simulink model "ControlMotor"  (R2024b)
settings: Solver=VariableStepAuto  StartTime=0.0  StopTime=inf  RelTol=1e-3
model workspace (MAT data in the model file):
  Speed = [255 255]
libraries: arduinolib x4
settings Model: Creator=m4ttn  LastModifiedBy=m4ttn

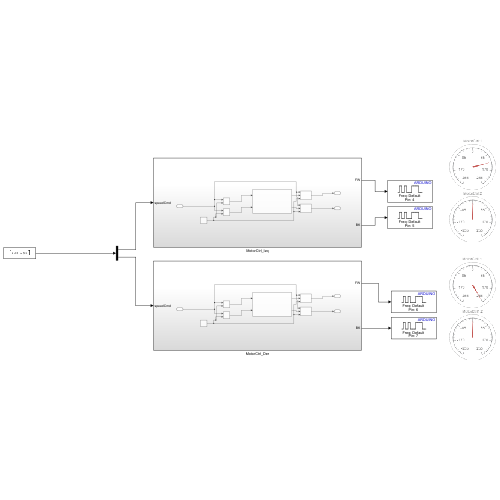
[thumbnail: Simulink's stored preview of the top-level diagram]
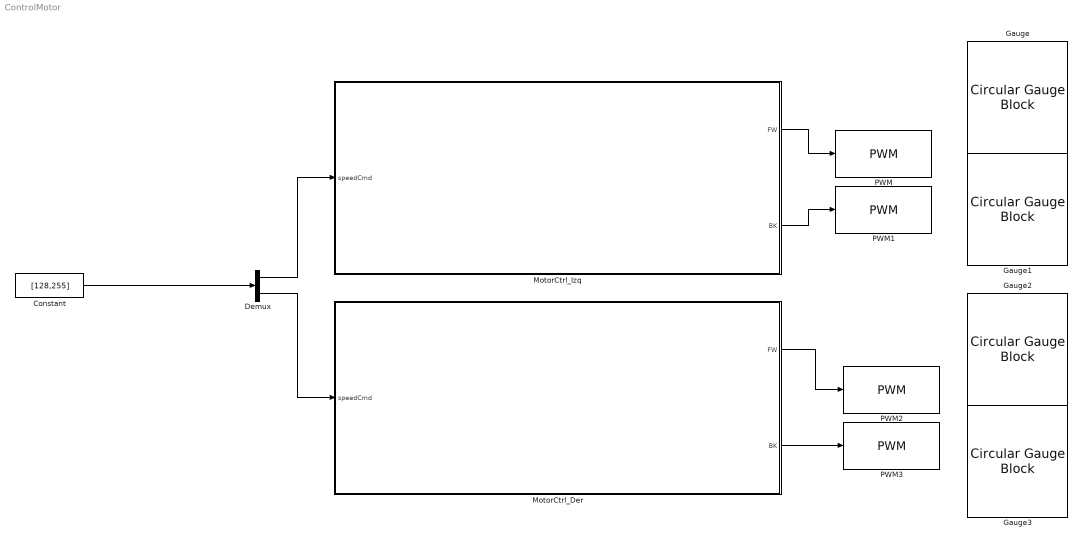
== system ControlMotor ==
  Constant : Constant  Value=[128,255]  OutDataTypeStr=int16
  Demux : Demux  Outputs=2
  Gauge{,1..3} (4 alike) : CircularGaugeBlock  ScaleMin=-255  ScaleMax=255
  MotorCtrl_Der : Subsystem
  MotorCtrl_Izq : Subsystem
  PWM : arduinolib/PWM  pinNumber=4  frequencyType=Default  desiredFrequency=490.2  achievableFrequency=490.2
  PWM1 : arduinolib/PWM  pinNumber=5  frequencyType=Default  desiredFrequency=490.2  achievableFrequency=490.2
  PWM2 : arduinolib/PWM  pinNumber=6  frequencyType=Default  desiredFrequency=490.2  achievableFrequency=490.2
  PWM3 : arduinolib/PWM  pinNumber=7  frequencyType=Default  desiredFrequency=490.2  achievableFrequency=490.2
  wires:
  Constant/1 -> Demux/1
  Demux/1 -> MotorCtrl_Izq/1(speedCmd)
  MotorCtrl_Izq/1(FW) -> PWM/1
  MotorCtrl_Izq/2(BK) -> PWM1/1
  Demux/2 -> MotorCtrl_Der/1(speedCmd)
  MotorCtrl_Der/1(FW) -> PWM2/1
  MotorCtrl_Der/2(BK) -> PWM3/1

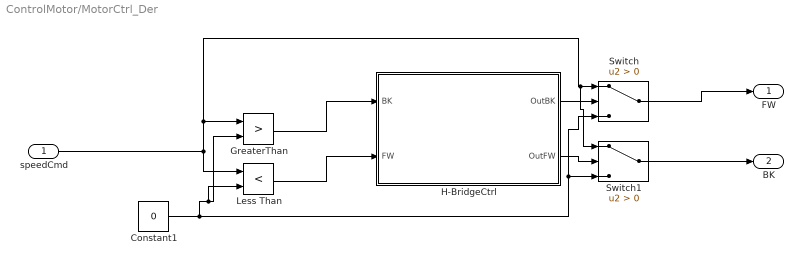
== system ControlMotor/MotorCtrl_Der ==
  speedCmd : Inport
  Constant1 : Constant  Value=0
  GreaterThan : RelationalOperator  Operator=>  OutDataTypeStr=boolean  RndMeth=Simplest  InputSameDT=off
  H-BridgeCtrl : Subsystem
  Less Than : RelationalOperator  Operator=<  OutDataTypeStr=boolean  RndMeth=Simplest  InputSameDT=off
  Switch : Switch  Criteria=u2 > Threshold  SaturateOnIntegerOverflow=off  InputSameDT=off
  Switch1 : Switch  Criteria=u2 > Threshold  SaturateOnIntegerOverflow=off  InputSameDT=off
  FW : Outport
  BK : Outport  Port=2
  wires:
  Less Than/1 -> H-BridgeCtrl/2(FW)
  H-BridgeCtrl/2(OutFW) -> Switch1/2
  speedCmd/1 -> GreaterThan/1, Switch1/1, Switch/1, Less Than/1
  H-BridgeCtrl/1(OutBK) -> Switch/2
  GreaterThan/1 -> H-BridgeCtrl/1(BK)
  Constant1/1 -> GreaterThan/2, Less Than/2, Switch/3, Switch1/3
  Switch/1 -> FW/1
  Switch1/1 -> BK/1

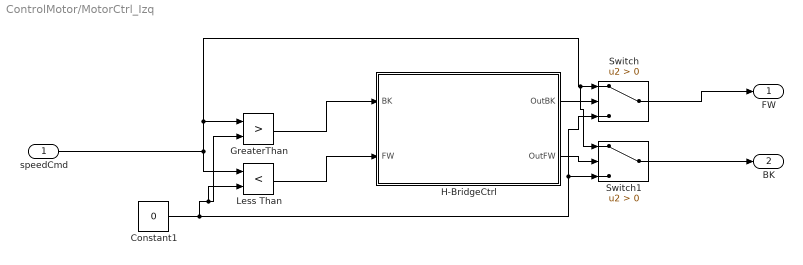
== system ControlMotor/MotorCtrl_Izq ==
  speedCmd : Inport
  Constant1 : Constant  Value=0
  GreaterThan : RelationalOperator  Operator=>  OutDataTypeStr=boolean  RndMeth=Simplest  InputSameDT=off
  H-BridgeCtrl : Subsystem
  Less Than : RelationalOperator  Operator=<  OutDataTypeStr=boolean  RndMeth=Simplest  InputSameDT=off
  Switch : Switch  Criteria=u2 > Threshold  SaturateOnIntegerOverflow=off  InputSameDT=off
  Switch1 : Switch  Criteria=u2 > Threshold  SaturateOnIntegerOverflow=off  InputSameDT=off
  FW : Outport
  BK : Outport  Port=2
  wires:
  Less Than/1 -> H-BridgeCtrl/2(FW)
  H-BridgeCtrl/2(OutFW) -> Switch1/2
  speedCmd/1 -> GreaterThan/1, Switch1/1, Switch/1, Less Than/1
  H-BridgeCtrl/1(OutBK) -> Switch/2
  GreaterThan/1 -> H-BridgeCtrl/1(BK)
  Constant1/1 -> GreaterThan/2, Less Than/2, Switch/3, Switch1/3
  Switch/1 -> FW/1
  Switch1/1 -> BK/1

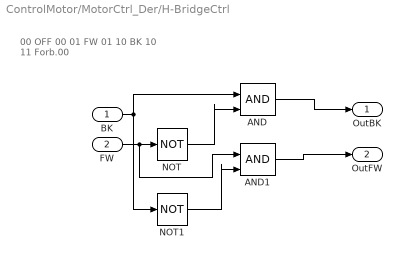
== system ControlMotor/MotorCtrl_Der/H-BridgeCtrl ==
  note: 00	OFF 00
      | 01   FW	 01
      | 10   BK	 10
      | 11   Forb.00
  BK : Inport
  FW : Inport  Port=2
  AND : Logic  IconShape=distinctive  AllPortsSameDT=off  OutDataTypeStr=boolean
  AND1 : Logic  IconShape=distinctive  AllPortsSameDT=off  OutDataTypeStr=boolean
  NOT : Logic  Operator=NOT  IconShape=distinctive  AllPortsSameDT=off  OutDataTypeStr=boolean
  NOT1 : Logic  Operator=NOT  IconShape=distinctive  AllPortsSameDT=off  OutDataTypeStr=boolean
  OutBK : Outport
  OutFW : Outport  Port=2
  wires:
  NOT/1 -> AND/2
  FW/1 -> AND1/1, NOT/1
  BK/1 -> NOT1/1, AND/1
  AND/1 -> OutBK/1
  NOT1/1 -> AND1/2
  AND1/1 -> OutFW/1

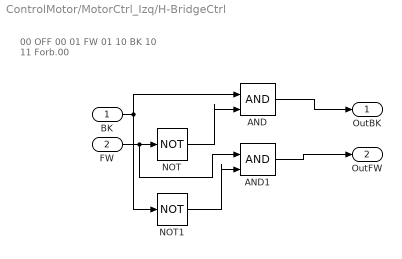
== system ControlMotor/MotorCtrl_Izq/H-BridgeCtrl ==
  note: 00	OFF 00
      | 01   FW	 01
      | 10   BK	 10
      | 11   Forb.00
  BK : Inport
  FW : Inport  Port=2
  AND : Logic  IconShape=distinctive  AllPortsSameDT=off  OutDataTypeStr=boolean
  AND1 : Logic  IconShape=distinctive  AllPortsSameDT=off  OutDataTypeStr=boolean
  NOT : Logic  Operator=NOT  IconShape=distinctive  AllPortsSameDT=off  OutDataTypeStr=boolean
  NOT1 : Logic  Operator=NOT  IconShape=distinctive  AllPortsSameDT=off  OutDataTypeStr=boolean
  OutBK : Outport
  OutFW : Outport  Port=2
  wires:
  NOT/1 -> AND/2
  FW/1 -> AND1/1, NOT/1
  BK/1 -> NOT1/1, AND/1
  AND/1 -> OutBK/1
  NOT1/1 -> AND1/2
  AND1/1 -> OutFW/1
